simulink model "PEMFuelCellSystem_Cathode_cEGR_Focused_v01"  (R2025b)
settings: Solver=VariableStepAuto  StartTime=0.0  StopTime=100  MaxStep=0.1  RelTol=1e-3  AbsTol=1e-3
model workspace (MAT data in the model file):
  Gas_properties_block = 'PEMFuelCellSystem_Before_v01/Anode_Hydrogen_BOP/Gas Mixture
Properties'
  Gas_properties_candidates : object (value not decoded)
  T_TLU = [223.15 228.15 233.15 238.15 243.15 248.15 253.15 258.15 263.15 268.15 272.66 273.15 ... (115 elements, 1x115)]
  anode_separator_D = 0.02
  anode_separator_T0 = 20
  anode_separator_area = 0.000314159265359
  anode_separator_dp_nominal = 0.0005
  anode_separator_extra_length = 0.04
  anode_separator_laminar_fraction = 0.001
  anode_separator_length = 0.12
  anode_separator_mdot_nominal = 0.01
  anode_separator_p0 = 0.101325
  anode_separator_roughness = 1.5e-05
  anode_tube_D = 0.02
  cathode_outlet_chamber_V = 0.2
  cathode_separator_D = 0.05
  cathode_separator_T0 = 20
  cathode_separator_area = 0.00196349540849
  cathode_separator_dp_nominal = 0.0005
  cathode_separator_extra_length = 0.05
  cathode_separator_laminar_fraction = 0.001
  cathode_separator_length = 0.15
  cathode_separator_mdot_nominal = 0.1
  cathode_separator_p0 = 0.101325
  cathode_separator_roughness = 1.5e-05
  cathode_tube_D = 0.05
  cegr_comp_map_t_denom_epsilon = 1e-09
  cegr_cond_tau = 1
  cegr_inlet_mixer_p0 = 0.101325
  cegr_outlet_chamber_p0 = 0.101325
  cegr_pipe_D = 0.05
  cegr_pipe_area = 0.00196349540849
  cegr_pipe_extra_length = 0.1
  cegr_pipe_length = 0.5
  cegr_pipe_p0 = 0.101325
  cegr_pipe_roughness = 1.5e-05
  cegr_valve_max_area = 0.000196349540849
  cegr_valve_open_min_area = 1e-10
  comp_inlet_mixer_V = 0.1
  comp_mdot_corr_TLU = [0 0 0 0 0 0.2 0.15 0.1 0.05 0 0.4 0.3 ... (15 elements, 5x3)]
  comp_p_ratio_TLU = [1 1.25 1.5 1.75 2]
  comp_rpm_TLU = [0 1800 3600]
  coolant_num_layers = 20
  coolant_num_passes = 12
  coolant_tube_D = 0.05
  coolant_w_channels = 1
  drive_cycle_current = [0 0 100 100]
  drive_cycle_power = [0 0 40 40]
  drive_cycle_time = [0 0.5 60.5 600]
  drive_cycle_voltage = [427.6 427.6 410 410]
  env_RH = 0.5
  env_T = 20
  env_p = 0.101325
  env_pSat_H2O = 0.00233931818334
  env_yH20 = 0.0115436377169
  env_yO2 = 0.21
  focused_anode_boundary_T_C = 20
  focused_anode_feed_p_MPa_abs = 0.3
  focused_anode_inlet_mdot_kg_s = 0.001
  focused_anode_inlet_p_MPa_abs = 0.161325
  focused_anode_outlet_p_MPa_abs = 0.101325
  focused_anode_pipe_area = 0.000314159265359
  focused_anode_pipe_extra_length = 0.1
  focused_anode_pipe_length = 1
  focused_anode_pipe_roughness = 1.5e-05
  focused_anode_yH2 = 0.9997
  focused_stack_temperature_C = 80
  humidifier_bypass_mode : string (value not decoded)
  intercooler_Dh = 0.05
  intercooler_T0 = 20
  intercooler_area = 0.00196349540849
  intercooler_cond_tau = 1
  intercooler_dp_nominal = 0.001
  intercooler_extra_length = 0.05
  intercooler_laminar_fraction = 0.001
  intercooler_length = 0.25
  intercooler_mdot_nominal = 0.1
  intercooler_p0 = 0.101325
  intercooler_roughness = 1.5e-05
  pSat_H2O_TLU = [0.0039376926592 0.00720321689378 0.0128411282011 0.0223441068076 0.0380050105363 0.0632733889962 0.103238678713 0.165273175188 0.259872929049 0.401739659013 0.586936061043 0.611151401419 ... (115 elements, 1x115)]
  pSat_TLU = [3379.45709837 5023.40410987 1277.63968517 0.0039376926592 3379.45809837 5023.40510987 1277.64068517 0.00720321689378 3379.45909837 5023.40610987 1277.64168517 0.0128411282011 ... (460 elements, 4x115)]
  radiator_H = 0.5
  radiator_L = 1
  radiator_N_fins = 12000
  radiator_N_tubes = 25
  radiator_W = 0.025
  radiator_air_area_fins = 11.5625
  radiator_air_area_primary = 1.223125
  radiator_cp = 910
  radiator_eta_fin = 0.7
  radiator_fin_spacing = 0.002
  radiator_gap_H = 0.0192708333333
  radiator_rho = 2700
  radiator_t_wall = 0.0001
  radiator_tube_H = 0.0015
  radiator_tube_Leq = 2.5
  routeA_air_control_mode_id = 2
  routeA_air_pid_Ki = 0.5
  routeA_air_pid_Kp = 5
  routeA_anode_inlet_pressure_MPa_abs = 0.161325
  routeA_anode_purge_enable = 1
  routeA_anode_purge_off_n2_mole_fraction = 0.1
  routeA_anode_purge_on_n2_mole_fraction = 0.5
  routeA_anode_recirculation_base_command = 0.2
  routeA_anode_recirculation_current_gain_A_inv = 0.00204081632653
  routeA_anode_rh_setpoint = 1
  routeA_backpressure_control_mode_id = 1
  routeA_cathode_humidifier_gain = 1
  routeA_cathode_rh_setpoint = 1
  routeA_cegr_enabled = 1
  routeA_cegr_valve_mode_id = 1
  routeA_command_profile = [0 0.5 60.5 600 0.101325 0.101325 0.101325 0.101325 20 20 20 20 ... (92 elements, 4x23)]
  routeA_command_profile_baseline = [0.101325 20 0.21 0.0115436377169 0.045 3 0.5 0.1613 1 1 0 70 ... (22 elements, 1x22)]
  routeA_command_profile_fields : string (value not decoded)
  routeA_command_profile_schema : string (value not decoded)
  routeA_current_default_ref_A = 28
  routeA_egr_control_Ki_area = 3.92699081699e-05
  routeA_egr_control_Kp_area = 0.000196349540849
  routeA_egr_control_mode_id = 1
  routeA_egr_target_input_mode_id = 1
  routeA_egr_valve_actuator_tau = 0.5
  routeA_egr_valve_area_direct = 3.92699081699e-06
  routeA_external_case_enabled = 0
  routeA_parameter_layer : string (value not decoded)
  routeA_stack_temperature_set_C = 80
  routeA_target_egr_ratio_comp_in = 0.02
  routeA_voltage_current_max_A = 392
  routeA_voltage_current_min_A = 0
  routeA_voltage_default_ref_V = 394.9
  routeA_voltage_pi_Ki = 0.05
  routeA_voltage_pi_Kp = 1
  separator_condensation_enabled = 1
  separator_l2_efficiency = 0.5
  separator_l2_source : string (value not decoded)
  stack_alpha = 0.7
  stack_area = 280
  stack_iL = 1.4
  stack_io = 0.0001
  stack_mea_cp = 870
  stack_mea_rho = 1800
  stack_num_cells = 400
  stack_num_channels = 8
  stack_t_gdl = 250
  stack_t_membrane = 125
  stack_w_channels = 1
  tank_T = 20
  tank_V = 120
  tank_p = 70
  tank_yH2 = 0.9997
libraries: FuelCell_lib x43, fl_lib x34, nesl_utility x33, slpidlib x4
(part 3 of 4)

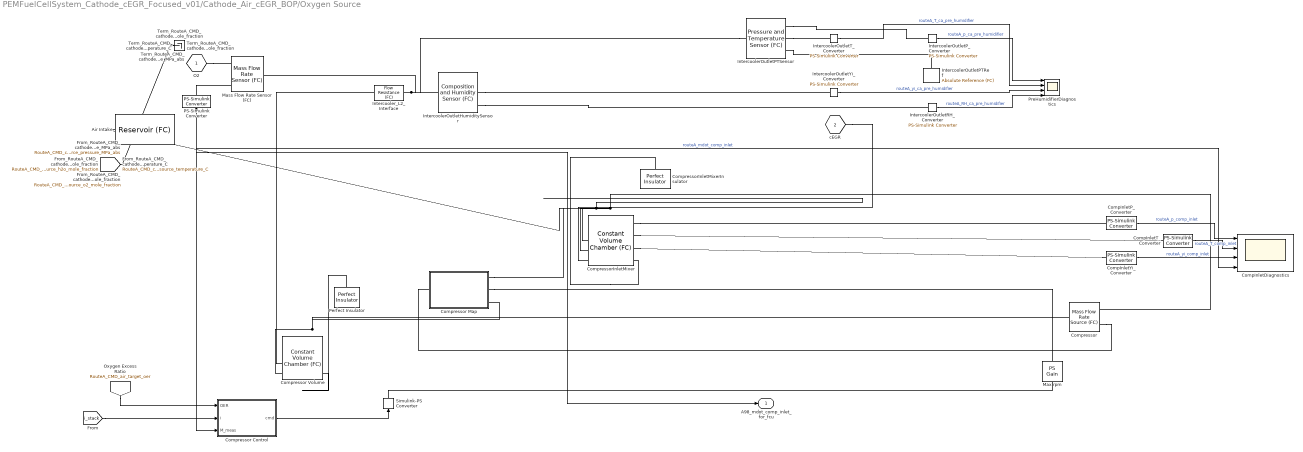
== system PEMFuelCellSystem_Cathode_cEGR_Focused_v01/Cathode_Air_cEGR_BOP/Oxygen Source ==
  Air Intake : FuelCell_lib/elements/Reservoir (FC)  constCond=true  p0=env_p MPa  T0=env_T degC  comp=FuelCell.enum.Composition.Mole  y0=[1-env_yO2-env_yH20; env_yO2; 0; env_yH20]  x0=[1; 0; 0; 0]  area=0.01 m^2
      settings: InternalSimscapePortConfiguration="{\"Bottom\":[],\"Left\":[],\"Right\":[],\"Top\":[{\"id\":\"A\",\"label\":\"A\",\"type\":\"FuelCell.FuelCell\"}]}"
  CompInletDiagnostics : Scope  NumInputPorts=4
  CompInletP_Converter : nesl_utility/PS-Simulink Converter  PhysicalDomain=network_engine_domain  SubClassName=ps_output  LeftPortType=input  RightPortType=output  PseudoPeriodic=off  Frequencies=[]  VectorFormat=inherit  Unit=inherit  AffineConversion=off
  CompInletT_Converter : nesl_utility/PS-Simulink Converter  PhysicalDomain=network_engine_domain  SubClassName=ps_output  LeftPortType=input  RightPortType=output  PseudoPeriodic=off  Frequencies=[]  VectorFormat=inherit  Unit=inherit  AffineConversion=off
  CompInletYi_Converter : nesl_utility/PS-Simulink Converter  PhysicalDomain=network_engine_domain  SubClassName=ps_output  LeftPortType=input  RightPortType=output  PseudoPeriodic=off  Frequencies=[]  VectorFormat=inherit  Unit=inherit  AffineConversion=off
  Compressor : FuelCell_lib/sources/Mass Flow Rate Source (FC)  source_type=foundation.enum.constant_controlled.controlled  flow_rate=0 kg/s  power_spec=foundation.enum.power_spec.isentropic  area_A=pi*cathode_tube_D^2/4 m^2  area_B=pi*cathode_tube_D^2/4 m^2  mdot_A_specify=off  mdot_A_priority=None  mdot_A=0.1 kg/s  mdot_A_nominal_specify=off  mdot_A_nominal_value=1  mdot_A_nominal_unit=kg/s  mdot_B_specify=off  mdot_B_priority=None  mdot_B=0.1 kg/s  mdot_B_nominal_specify=off  mdot_B_nominal_value=1  mdot_B_nominal_unit=kg/s  phi_A_specify=off  phi_A_priority=None  phi_A=0 J/s  phi_A_nominal_specify=off  phi_A_nominal_value=1  phi_A_nominal_unit=J/s  phi_B_specify=off  phi_B_priority=None  phi_B=0 J/s  phi_B_nominal_specify=off  phi_B_nominal_value=1  phi_B_nominal_unit=J/s  mdot_A_i_specify=off  mdot_A_i_priority=None  mdot_A_i=[0; 0; 0; 0] kg/s  mdot_A_i_nominal_specify=off  mdot_A_i_nominal_value=1  mdot_A_i_nominal_unit=kg/s  mdot_B_i_specify=off  mdot_B_i_priority=None  mdot_B_i=[0; 0; 0; 0] kg/s  mdot_B_i_nominal_specify=off  mdot_B_i_nominal_value=1  mdot_B_i_nominal_unit=kg/s
      settings: InternalSimscapePortConfiguration="{\"Bottom\":[],\"Left\":[{\"id\":\"M\",\"label\":\"M\",\"type\":\"input\"},{\"id\":\"A\",\"label\":\"A\",\"type\":\"FuelCell.FuelCell\"}],\"Right\":[{\"id\":\"B\",\"label\":\"B\",\"type\":\"FuelCell.FuelCell\"}],\"Top\":[]}"
  Compressor Volume : FuelCell_lib/elements/Constant Volume Chamber (FC)  V0=0.3 l  num_ports=foundation.enum.num_ports.two  area_A=pi*cathode_tube_D^2/4 m^2  area_B=pi*cathode_tube_D^2/4 m^2  area_C=0.01 m^2  area_D=0.01 m^2  cond_spec=FuelCell.enum.ChamberCondSpec.Enabled  tau_c=1e-3 s  is_cond=[0; 0; 0; 0]  out_comp=FuelCell.enum.Composition.Mole  p0=env_p MPa  T0=env_T degC  comp=FuelCell.enum.Composition.Mole  y0=[1-env_yO2-env_yH20; env_yO2; 0; env_yH20]  x0=[1; 0; 0; 0]
      settings: InternalSimscapePortConfiguration="{\"Bottom\":[{\"id\":\"H\",\"label\":\"H\",\"type\":\"foundation.thermal.thermal\"}],\"Left\":[{\"id\":\"MIn\",\"label\":\"MIn\",\"type\":\"input\"},{\"id\":\"TIn\",\"label\":\"TIn\",\"type\":\"input\"}],\"Right\":[{\"id\":\"pC\",\"label\":\"p\",\"type\":\"output\"},{\"id\":\"TC\",\"label\":\"T\",\"type\":\"output\"},{\"id\":\"yC_i\",\"label\":\"y_i\",\"type\":\"output\"}],\"Top\":[{\"id\":\"A\",\"label\":\"A\",\"type\":\"FuelCell.FuelCell\"},{\"id\":\"B\",\"label\":\"B\",\"type\":\"FuelCell.FuelCell\"}]}"
  Compressor Control : Subsystem
  Compressor Map : Subsystem
  CompressorInletMixer : FuelCell_lib/elements/Constant Volume Chamber (FC)  V0=comp_inlet_mixer_V l  num_ports=foundation.enum.num_ports.three  area_A=cegr_pipe_area m^2  area_B=cegr_pipe_area m^2  area_C=cegr_pipe_area m^2  area_D=0.01 m^2  cond_spec=FuelCell.enum.ChamberCondSpec.Enabled  tau_c=cegr_cond_tau s  is_cond=[0; 0; 0; 1]  out_comp=FuelCell.enum.Composition.Mole  p0=cegr_inlet_mixer_p0 MPa  T0=env_T degC  comp=FuelCell.enum.Composition.Mole  y0=[1-env_yO2-env_yH20; env_yO2; 0; env_yH20]  x0=[1; 0; 0; 0]
      settings: InternalSimscapePortConfiguration="{\"Bottom\":[{\"id\":\"H\",\"label\":\"H\",\"type\":\"foundation.thermal.thermal\"}],\"Left\":[{\"id\":\"MIn\",\"label\":\"MIn\",\"type\":\"input\"},{\"id\":\"TIn\",\"label\":\"TIn\",\"type\":\"input\"}],\"Right\":[{\"id\":\"pC\",\"label\":\"p\",\"type\":\"output\"},{\"id\":\"TC\",\"label\":\"T\",\"type\":\"output\"},{\"id\":\"yC_i\",\"label\":\"y_i\",\"type\":\"output\"}],\"Top\":[{\"id\":\"A\",\"label\":\"A\",\"type\":\"FuelCell.FuelCell\"},{\"id\":\"B\",\"label\":\"B\",\"type\":\"FuelCell.FuelCell\"},{\"id\":\"C\",\"label\":\"C\",\"type\":\"FuelCell.FuelCell\"}]}"
  CompressorInletMixerInsulator : fl_lib/Thermal/Thermal Elements/Perfect Insulator  T_specify=off  T_priority=None  T=env_T degC  T_nominal_specify=off  T_nominal_value=1  T_nominal_unit=K
  IntercoolerOutletHumiditySensor : FuelCell_lib/sensors/Composition and Humidity Sensor (FC)
      settings: InternalSimscapePortConfiguration="{\"Bottom\":[],\"Left\":[{\"id\":\"A\",\"label\":\"A\",\"type\":\"FuelCell.FuelCell\"}],\"Right\":[{\"id\":\"x_i\",\"label\":\"x_i\",\"type\":\"output\"},{\"id\":\"y_i\",\"label\":\"y_i\",\"type\":\"output\"},{\"id\":\"W\",\"label\":\"W\",\"type\":\"output\"}],\"Top\":[]}"
  IntercoolerOutletPTRef : FuelCell_lib/elements/Absolute Reference (FC)
      settings: InternalSimscapePortConfiguration="{\"Bottom\":[],\"Left\":[{\"id\":\"A\",\"label\":\"\",\"type\":\"FuelCell.FuelCell\"}],\"Right\":[],\"Top\":[]}"
  IntercoolerOutletPTSensor : FuelCell_lib/sensors/Pressure and Temperature Sensor (FC)
      settings: InternalSimscapePortConfiguration="{\"Bottom\":[],\"Left\":[{\"id\":\"A\",\"label\":\"A\",\"type\":\"FuelCell.FuelCell\"}],\"Right\":[{\"id\":\"P\",\"label\":\"P\",\"type\":\"output\"},{\"id\":\"T\",\"label\":\"T\",\"type\":\"output\"},{\"id\":\"B\",\"label\":\"B\",\"type\":\"FuelCell.FuelCell\"}],\"Top\":[]}"
  IntercoolerOutletP_Converter : nesl_utility/PS-Simulink Converter  PhysicalDomain=network_engine_domain  SubClassName=ps_output  LeftPortType=input  RightPortType=output  PseudoPeriodic=off  Frequencies=[]  VectorFormat=inherit  Unit=inherit  AffineConversion=off
  IntercoolerOutletRH_Converter : nesl_utility/PS-Simulink Converter  PhysicalDomain=network_engine_domain  SubClassName=ps_output  LeftPortType=input  RightPortType=output  PseudoPeriodic=off  Frequencies=[]  VectorFormat=inherit  Unit=inherit  AffineConversion=off
  IntercoolerOutletT_Converter : nesl_utility/PS-Simulink Converter  PhysicalDomain=network_engine_domain  SubClassName=ps_output  LeftPortType=input  RightPortType=output  PseudoPeriodic=off  Frequencies=[]  VectorFormat=inherit  Unit=inherit  AffineConversion=off
  IntercoolerOutletYi_Converter : nesl_utility/PS-Simulink Converter  PhysicalDomain=network_engine_domain  SubClassName=ps_output  LeftPortType=input  RightPortType=output  PseudoPeriodic=off  Frequencies=[]  VectorFormat=inherit  Unit=inherit  AffineConversion=off
  Intercooler_L2_Interface : FuelCell_lib/elements/Flow Resistance (FC)  var_res=false  delta_p_nominal=intercooler_dp_nominal MPa  mdot_nominal=intercooler_mdot_nominal kg/s  rho_nominal=0 kg/m^3  laminar_fraction=intercooler_laminar_fraction  area=intercooler_area m^2  leak_thresh=1e-5
      settings: InternalSimscapePortConfiguration="{\"Bottom\":[],\"Left\":[{\"id\":\"A\",\"label\":\"A\",\"type\":\"FuelCell.FuelCell\"}],\"Right\":[{\"id\":\"B\",\"label\":\"B\",\"type\":\"FuelCell.FuelCell\"}],\"Top\":[]}"
  Mass Flow Rate Sensor (FC) : FuelCell_lib/sensors/Mass Flow Rate Sensor (FC)
      settings: InternalSimscapePortConfiguration="{\"Bottom\":[],\"Left\":[{\"id\":\"A\",\"label\":\"A\",\"type\":\"FuelCell.FuelCell\"}],\"Right\":[{\"id\":\"M\",\"label\":\"M\",\"type\":\"output\"},{\"id\":\"Phi_out\",\"label\":\"Phi\",\"type\":\"output\"},{\"id\":\"M_i\",\"label\":\"M_i\",\"type\":\"output\"},{\"id\":\"B\",\"label\":\"B\",\"type\":\"FuelCell.FuelCell\"}],\"Top\":[]}"
  Max rpm : fl_lib/Physical Signals/Functions/PS Gain  gain=max(comp_rpm_TLU) rpm
  PS-Simulink Converter : nesl_utility/PS-Simulink Converter  PhysicalDomain=network_engine_domain  SubClassName=ps_output  LeftPortType=input  RightPortType=output  PseudoPeriodic=off  Frequencies=[]  VectorFormat=1-D array  Unit=kg/s  AffineConversion=off
  Perfect Insulator : fl_lib/Thermal/Thermal Elements/Perfect Insulator  T_specify=off  T_priority=None  T=env_T degC  T_nominal_specify=off  T_nominal_value=1  T_nominal_unit=K
  PreHumidifierDiagnostics : Scope  NumInputPorts=4
  Simulink-PS Converter : nesl_utility/Simulink-PS Converter  PhysicalDomain=network_engine_domain  SubClassName=ps_input  LeftPortType=input  RightPortType=output  PseudoPeriodic=off  Frequencies=[]  NoiseDistribution=none  NoiseParameters=[]  Unit=1  AffineConversion=off  FilteringAndDerivatives=provide  SimscapeFilterOrder=1  InputFilterTimeConstant=0.001  UdotUserProvided=0
  Term_RouteA_CMD_cathode_source_h2o_mole_fraction : Terminator
  Term_RouteA_CMD_cathode_source_o2_mole_fraction : Terminator
  Term_RouteA_CMD_cathode_source_pressure_MPa_abs : Terminator
  Term_RouteA_CMD_cathode_source_temperature_C : Terminator
  O2 : PMIOPort  Side=Left
  cEGR : PMIOPort  Port=2  Side=Left
  A98_mdot_comp_inlet_for_fcu : Outport
  wires:
  CompInletT_Converter/1 -> CompInletDiagnostics/2  "routeA_T_comp_inlet"
  CompInletP_Converter/1 -> CompInletDiagnostics/1  "routeA_p_comp_inlet"
  Compressor Control/1(cmd) -> Simulink-PS Converter/1
  [i_stack] -> Compressor Control/2(i)
  CompInletYi_Converter/1 -> CompInletDiagnostics/3  "routeA_yi_comp_inlet"
  PS-Simulink Converter/1 -> A98_mdot_comp_inlet_for_fcu/1, Compressor Control/3(M_meas), CompInletDiagnostics/4  "routeA_mdot_comp_inlet"
  IntercoolerOutletP_Converter/1 -> PreHumidifierDiagnostics/1  "routeA_p_ca_pre_humidifier"
  IntercoolerOutletT_Converter/1 -> PreHumidifierDiagnostics/2  "routeA_T_ca_pre_humidifier"
  IntercoolerOutletYi_Converter/1 -> PreHumidifierDiagnostics/3  "routeA_yi_ca_pre_humidifier"
  IntercoolerOutletRH_Converter/1 -> PreHumidifierDiagnostics/4  "routeA_RH_ca_pre_humidifier"
  [RouteA_CMD_air_target_oer] -> Compressor Control/1(OER)
  [RouteA_CMD_cathode_source_o2_mole_fraction] -> Term_RouteA_CMD_cathode_source_o2_mole_fraction/1
  [RouteA_CMD_cathode_source_h2o_mole_fraction] -> Term_RouteA_CMD_cathode_source_h2o_mole_fraction/1
  [RouteA_CMD_cathode_source_pressure_MPa_abs] -> Term_RouteA_CMD_cathode_source_pressure_MPa_abs/1
  [RouteA_CMD_cathode_source_temperature_C] -> Term_RouteA_CMD_cathode_source_temperature_C/1
  connections:
  CompressorInletMixer/LConn3 -- Air Intake/LConn1
  IntercoolerOutletHumiditySensor/RConn3 -- IntercoolerOutletRH_Converter/LConn1
  IntercoolerOutletHumiditySensor/RConn2 -- IntercoolerOutletYi_Converter/LConn1
  IntercoolerOutletPTSensor/RConn2 -- IntercoolerOutletT_Converter/LConn1
  IntercoolerOutletPTSensor/RConn1 -- IntercoolerOutletP_Converter/LConn1
  IntercoolerOutletPTSensor/LConn1 -- Intercooler_L2_Interface/RConn1 -- Mass Flow Rate Sensor (FC)/LConn1 -- IntercoolerOutletHumiditySensor/LConn1
  Compressor/LConn1 -- Compressor Map/LConn1
  CompressorInletMixer/RConn2 -- CompInletT_Converter/LConn1
  CompressorInletMixer/RConn1 -- CompInletP_Converter/LConn1
  Compressor Map/RConn2 -- Max rpm/RConn1
  CompressorInletMixer/LConn4 -- Compressor Map/RConn1 -- Compressor/LConn2
  cEGR/RConn1 -- CompressorInletMixer/LConn5
  Simulink-PS Converter/RConn1 -- Max rpm/LConn1
  CompressorInletMixer/RConn3 -- CompInletYi_Converter/LConn1
  Compressor Map/RConn3 -- Compressor Volume/LConn4 -- Compressor/RConn1
  CompressorInletMixerInsulator/LConn1 -- CompressorInletMixer/RConn4
  Perfect Insulator/LConn1 -- Compressor Volume/RConn4
  PS-Simulink Converter/LConn1 -- Mass Flow Rate Sensor (FC)/RConn1
  O2/RConn1 -- Mass Flow Rate Sensor (FC)/RConn4
  IntercoolerOutletPTSensor/RConn3 -- IntercoolerOutletPTRef/LConn1
  Intercooler_L2_Interface/LConn1 -- Compressor Volume/LConn3

== system PEMFuelCellSystem_Cathode_cEGR_Focused_v01/Cathode_Exhaust_Backpressure_Water/Cathode Exhaust ==
  Constant1 : Constant  Value=0
  Convective Heat Transfer1 : fl_lib/Thermal/Thermal Elements/Convective Heat Transfer  thermal_type=foundation.enum.constant_variable.constant  area=pi*cathode_tube_D*1 m^2  heat_tr_coeff=20 W/(m^2 * K)  min_heat_tr_coeff=1e-3 W/(K*m^2)  T_specify=off  T_priority=None  T=0 K  T_nominal_specify=off  T_nominal_value=1  T_nominal_unit=K  Q_specify=off  Q_priority=None  Q=0 W  Q_nominal_specify=off  Q_nominal_value=1  Q_nominal_unit=W
  Environment : FuelCell_lib/elements/Reservoir (FC)  constCond=true  p0=env_p MPa  T0=env_T degC  comp=FuelCell.enum.Composition.Mole  y0=[1-env_yO2-env_yH20; env_yO2; 0; env_yH20]  x0=[1; 0; 0; 0]  area=pi*cathode_tube_D^2/4 m^2
      settings: InternalSimscapePortConfiguration="{\"Bottom\":[],\"Left\":[],\"Right\":[],\"Top\":[{\"id\":\"A\",\"label\":\"A\",\"type\":\"FuelCell.FuelCell\"}]}"
  Environment Temperature : fl_lib/Thermal/Thermal Sources/Temperature Source  temperature=env_T degC
  Pipe (N Gas)1 : FuelCell_lib/elements/Pipe (FC)  length=1 m  area=pi*cathode_tube_D^2/4 m^2  Dh=cathode_tube_D m  extra_length=0.1 m  roughness=15e-6 m  Re_lam=2000  Re_tur=4000  shape_factor=64  Nu_lam=3.66  tau_c=1e-3 s  isCond=[0; 0; 0; 0]  volMeas=false  compMeas=FuelCell.enum.Composition.Mole  p0=env_p MPa  T0=env_T degC  comp=FuelCell.enum.Composition.Mole  y0=[1-env_yO2-env_yH20; env_yO2; 0; env_yH20]  x0=[1; 0; 0; 0]
      settings: InternalSimscapePortConfiguration="{\"Bottom\":[{\"id\":\"MIn\",\"label\":\"M_in\",\"type\":\"input\"},{\"id\":\"TIn\",\"label\":\"T_in\",\"type\":\"input\"}],\"Left\":[{\"id\":\"A\",\"label\":\"A\",\"type\":\"FuelCell.FuelCell\"},{\"id\":\"H\",\"label\":\"H\",\"type\":\"foundation.thermal.thermal\"}],\"Right\":[{\"id\":\"B\",\"label\":\"B\",\"type\":\"FuelCell.FuelCell\"}],\"Top\":[]}"
  Pressure Relief Valve : Subsystem  Tag=PublishSubsystem  mask(Pressure Relief Valve){D=cathode_tube_D, r_min=1e-4, r_max=0.8, p_range=0.005}
      mask prompts: D "Connecting tube diameter (m)"; r_min "Min diameter ratio"; r_max "Max diameter ratio"; p_range "Pressure regulation range (MPa)"
      mask help: This subsystem models a pressure relief valve that maintains a set pressure at port A. The valve is normally closed. When the pressure is above the set pressure, it begins to open.
  Simulink-PS Converter1 : nesl_utility/Simulink-PS Converter  PhysicalDomain=network_engine_domain  SubClassName=ps_input  LeftPortType=input  RightPortType=output  PseudoPeriodic=off  Frequencies=[]  NoiseDistribution=none  NoiseParameters=[]  Unit=MPa  AffineConversion=off  FilteringAndDerivatives=provide  SimscapeFilterOrder=1  InputFilterTimeConstant=0.001  UdotUserProvided=0
  Sum : Sum  Inputs=++|
  C : PMIOPort  Side=Left
  wires:
  Sum/1 -> Simulink-PS Converter1/1
  Constant1/1 -> Sum/2
  [RouteA_CMD_cathode_outlet_pressure_MPa_abs] -> Sum/1
  connections:
  C/RConn1 -- Pipe (N Gas)1/LConn1
  Simulink-PS Converter1/RConn1 -- Pressure Relief Valve/LConn2
  Pipe (N Gas)1/RConn1 -- Pressure Relief Valve/LConn1
  Pressure Relief Valve/RConn1 -- Environment/LConn1
  Convective Heat Transfer1/LConn1 -- Pipe (N Gas)1/LConn2
  Environment Temperature/LConn1 -- Convective Heat Transfer1/RConn1

== system PEMFuelCellSystem_Cathode_cEGR_Focused_v01/Stack_Core/Anode Gas Channels ==
  Anode : FuelCell_lib/elements/Constant Volume Chamber (FC)  V0=stack_w_channels^2 * stack_num_channels * stack_num_cells * sqrt(stack_area) cm^3  num_ports=foundation.enum.num_ports.three  area_A=stack_w_channels^2 * stack_num_channels * stack_num_cells cm^2  area_B=stack_w_channels^2 * stack_num_channels * stack_num_cells cm^2  area_C=stack_w_channels^2 * stack_num_channels * stack_num_cells cm^2  area_D=0.01 m^2  cond_spec=FuelCell.enum.ChamberCondSpec.Enabled  tau_c=1e-3 s  is_cond=[0; 0; 0; 0]  out_comp=FuelCell.enum.Composition.Mass  p0=env_p MPa  T0=env_T degC  comp=FuelCell.enum.Composition.Mole  y0=[0; 0; 1; 0]  x0=[1; 0; 0; 0]
      settings: InternalSimscapePortConfiguration="{\"Bottom\":[{\"id\":\"H\",\"label\":\"H\",\"type\":\"foundation.thermal.thermal\"}],\"Left\":[{\"id\":\"MIn\",\"label\":\"MIn\",\"type\":\"input\"},{\"id\":\"TIn\",\"label\":\"TIn\",\"type\":\"input\"}],\"Right\":[{\"id\":\"pC\",\"label\":\"p\",\"type\":\"output\"},{\"id\":\"TC\",\"label\":\"T\",\"type\":\"output\"},{\"id\":\"xC_i\",\"label\":\"x_i\",\"type\":\"output\"}],\"Top\":[{\"id\":\"A\",\"label\":\"A\",\"type\":\"FuelCell.FuelCell\"},{\"id\":\"B\",\"label\":\"B\",\"type\":\"FuelCell.FuelCell\"},{\"id\":\"C\",\"label\":\"C\",\"type\":\"FuelCell.FuelCell\"}]}"
  A : PMIOPort  Side=Right
  Min : PMIOPort  Port=2  Side=Right
  Tin : PMIOPort  Port=3  Side=Right
  H : PMIOPort  Port=4  Side=Right
  B : PMIOPort  Port=5  Side=Left
  C : PMIOPort  Port=6  Side=Left
  xi : PMIOPort  Port=7  Side=Left
  connections:
  B/RConn1 -- Anode/LConn4
  Min/RConn1 -- Anode/LConn1
  Tin/RConn1 -- Anode/LConn2
  xi/RConn1 -- Anode/RConn3
  Anode/LConn5 -- C/RConn1
  A/RConn1 -- Anode/LConn3
  H/RConn1 -- Anode/RConn4

== system PEMFuelCellSystem_Cathode_cEGR_Focused_v01/Stack_Core/Cathode Gas Channels ==
  Cathode : FuelCell_lib/elements/Constant Volume Chamber (FC)  V0=stack_w_channels^2 * stack_num_channels * stack_num_cells * sqrt(stack_area) cm^3  num_ports=foundation.enum.num_ports.three  area_A=stack_w_channels^2 * stack_num_channels * stack_num_cells cm^2  area_B=stack_w_channels^2 * stack_num_channels * stack_num_cells cm^2  area_C=stack_w_channels^2 * stack_num_channels * stack_num_cells cm^2  area_D=0.01 m^2  cond_spec=FuelCell.enum.ChamberCondSpec.Enabled  tau_c=1e-3 s  is_cond=[0; 0; 0; 0]  out_comp=FuelCell.enum.Composition.Mass  p0=env_p MPa  T0=env_T degC  comp=FuelCell.enum.Composition.Mole  y0=[1-env_yO2-env_yH20; env_yO2; 0; env_yH20]  x0=[1; 0; 0; 0]
      settings: InternalSimscapePortConfiguration="{\"Bottom\":[{\"id\":\"H\",\"label\":\"H\",\"type\":\"foundation.thermal.thermal\"}],\"Left\":[{\"id\":\"MIn\",\"label\":\"MIn\",\"type\":\"input\"},{\"id\":\"TIn\",\"label\":\"TIn\",\"type\":\"input\"}],\"Right\":[{\"id\":\"pC\",\"label\":\"p\",\"type\":\"output\"},{\"id\":\"TC\",\"label\":\"T\",\"type\":\"output\"},{\"id\":\"xC_i\",\"label\":\"x_i\",\"type\":\"output\"}],\"Top\":[{\"id\":\"A\",\"label\":\"A\",\"type\":\"FuelCell.FuelCell\"},{\"id\":\"B\",\"label\":\"B\",\"type\":\"FuelCell.FuelCell\"},{\"id\":\"C\",\"label\":\"C\",\"type\":\"FuelCell.FuelCell\"}]}"
  A : PMIOPort  Side=Right
  Min : PMIOPort  Port=2  Side=Right
  Tin : PMIOPort  Port=3  Side=Right
  H : PMIOPort  Port=4  Side=Right
  B : PMIOPort  Port=5  Side=Left
  C : PMIOPort  Port=6  Side=Left
  xi : PMIOPort  Port=7  Side=Left
  connections:
  B/RConn1 -- Cathode/LConn4
  Min/RConn1 -- Cathode/LConn1
  Tin/RConn1 -- Cathode/LConn2
  xi/RConn1 -- Cathode/RConn3
  H/RConn1 -- Cathode/RConn4
  Cathode/LConn5 -- C/RConn1
  A/RConn1 -- Cathode/LConn3

== system PEMFuelCellSystem_Cathode_cEGR_Focused_v01/System_Control_Observability/Electrical Load ==
  Controlled Current Source : fl_lib/Electrical/Electrical Sources/Controlled Current Source
  Electrical Reference : fl_lib/Electrical/Electrical Elements/Electrical Reference
  Inputs : Subsystem  Variant=on  VariantControlMode=label  LabelModeActiveChoice=Voltage
      settings: PortSchema="{\"entries\":[{\"content\":{\"sides\":[{\"content\":{\"connectorIds\":[\"LConn1\"]},\"type\":\"ConnectorPlacement.EquallySpacedRectSide\",\"uuid\":\"316ab41f-9548-4c29-941b-82cd3006a9cc\"},{\"content\":{\"connectorIds\":[],\"side\":\"RIGHT\"},\"type\":\"ConnectorPlacement.EquallySpacedRectSide\",\"uuid\":\"21ddf6a1-5f8a-47a4-ab15-3c27c3a556ce\"},{\"content\":{\"connectorIds\":[\"LConn2\"],\"side\":\"TOP\"},\"type\":\"ConnectorPlacement.EquallySpacedRectSide\",\"uuid\":\"59191a52-f145-4ac2-9cf2-0e0b54b3d2a8\"}]},\"type\":\"ConnectorPlacement.EquallySpacedConnector\",\"uuid\":\"e8f988fd-b412-4b1a-aaea-374cf82170cc\"}],\"packageUris\":[\"http://schema.mathworks.com/mf0/Connector/R2020b\"],\"version\":\"1.0\"}"
      mask Display:
      | blk = get_param(gcb, 'CompiledActiveChoiceBlock');
      | eval(get_param(blk, 'MaskDisplay'))
  Voltage Sensor : fl_lib/Electrical/Electrical Sensors/Voltage Sensor
  - : PMIOPort  Side=Right
  + : PMIOPort  Port=2  Side=Right
  connections:
  Electrical Reference/LConn1 -- Controlled Current Source/LConn1 -- -/RConn1 -- Voltage Sensor/RConn2
  +/RConn1 -- Voltage Sensor/LConn1 -- Controlled Current Source/RConn2
  Voltage Sensor/RConn1 -- Inputs/LConn2
  Inputs/LConn1 -- Controlled Current Source/RConn1

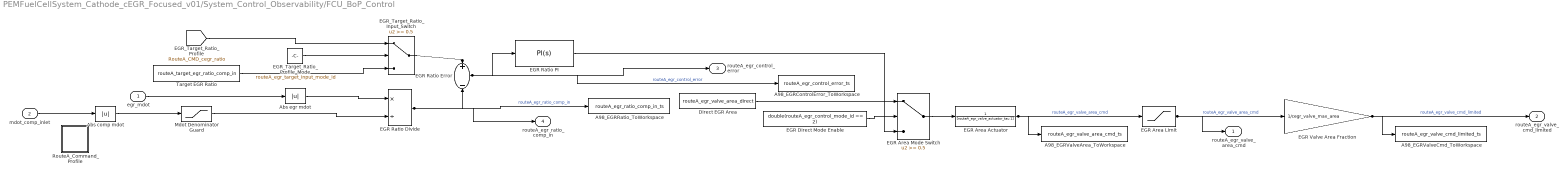
== system PEMFuelCellSystem_Cathode_cEGR_Focused_v01/System_Control_Observability/FCU_BoP_Control ==
  egr_mdot : Inport
  mdot_comp_inlet : Inport  Port=2
  A98_EGRControlError_ToWorkspace : ToWorkspace  VariableName=routeA_egr_control_error_ts  SaveFormat=Timeseries  SampleTime=-1
  A98_EGRRatio_ToWorkspace : ToWorkspace  VariableName=routeA_egr_ratio_comp_in_ts  SaveFormat=Timeseries  SampleTime=-1
  A98_EGRValveArea_ToWorkspace : ToWorkspace  VariableName=routeA_egr_valve_area_cmd_ts  SaveFormat=Timeseries  SampleTime=-1
  A98_EGRValveCmd_ToWorkspace : ToWorkspace  VariableName=routeA_egr_valve_cmd_limited_ts  SaveFormat=Timeseries  SampleTime=-1
  Abs comp mdot : Abs  ZeroCross=off  SaturateOnIntegerOverflow=off
  Abs egr mdot : Abs  ZeroCross=off  SaturateOnIntegerOverflow=off
  Direct EGR Area : Constant  Value=routeA_egr_valve_area_direct
  EGR Area Actuator : TransferFcn  Denominator=[routeA_egr_valve_actuator_tau 1]
  EGR Area Limit : Saturate  UpperLimit=cegr_valve_max_area  LowerLimit=cegr_valve_open_min_area
  EGR Area Mode Switch : Switch  Threshold=0.5  SaturateOnIntegerOverflow=off  InputSameDT=off
  EGR Direct Mode Enable : Constant  Value=double(routeA_egr_control_mode_id == 2)
  EGR Ratio Divide : Product  Inputs=*/
  EGR Ratio Error : Sum  Inputs=+-
  EGR Ratio PI : slpidlib/PID Controller  Controller=PI  Form=Parallel  TimeDomain=Continuous-time  UseExternalTs=off  SampleTime=-1  IntegratorMethod=Forward Euler  FilterMethod=Forward Euler  ControllerParametersSource=internal  P=routeA_egr_control_Kp_area  I=routeA_egr_control_Ki_area  UseKiTs=off  D=0  UseExternalDerivativeSource=off  N=100  UseFilter=on  TunerSelectOption=Transfer Function Based (PID Tuner App)  ZeroCross=off  InitialConditionSource=internal  InitialConditionForIntegrator=cegr_valve_open_min_area  InitialConditionForFilter=0  DifferentiatorICPrevScaledInput=0  ExternalReset=none  TrackingMode=off  Kt=1  LimitOutput=on  SatLimitsSource=internal  UpperSaturationLimit=cegr_valve_max_area  LowerSaturationLimit=cegr_valve_open_min_area  LinearizeAsGain=on  AntiWindupMode=none  Kb=1  LimitIntegrator=off  UpperIntegratorSaturationLimit=inf  LowerIntegratorSaturationLimit=-inf  POutMin=[]  POutMax=[]  IOutMin=[]  IOutMax=[]  DOutMin=[]  DOutMax=[]  NOutMin=[]  NOutMax=[]  SumOutMin=[]  SumOutMax=[]  SaturationOutMin=[]  SaturationOutMax=[]  PParamMin=[]  PParamMax=[]  IParamMin=[]  IParamMax=[]  DParamMin=[]  DParamMax=[]  NParamMin=[]  NParamMax=[]  KbParamMin=[]  KbParamMax=[]  KtParamMin=[]  KtParamMax=[]  KbOutMin=[]  KbOutMax=[]  KtOutMin=[]  KtOutMax=[]  IntegratorOutMin=[]  IntegratorOutMax=[]  FilterOutMin=[]  FilterOutMax=[]  SumI1OutMin=[]  SumI1OutMax=[]  SumI2OutMin=[]  SumI2OutMax=[]  SumI3OutMin=[]  SumI3OutMax=[]  SumI4OutMin=[]  SumI4OutMax=[]  SumDOutMin=[]  SumDOutMax=[]  DifferentiatorOutMin=[]  DifferentiatorOutMax=[]  FilterDiffOutCoefMin=[]  FilterDiffOutCoefMax=[]  ReciprocalOutMin=[]  ReciprocalOutMax=[]  SumDenOutMin=[]  SumDenOutMax=[]  SumNumOutMin=[]  SumNumOutMax=[]  DivideOutMin=[]  DivideOutMax=[]  UdiffTsProdOutMin=[]  UdiffTsProdOutMax=[]  NTsProdOutMin=[]  NTsProdOutMax=[]  UintegralTsProdOutMin=[]  UintegralTsProdOutMax=[]  UngainTsProdOutMin=[]  UngainTsProdOutMax=[]  ClampingZeroOutDataTypeStr=Inherit: Inherit via back propagation  ClampingZeroOutMin=[]  ClampingZeroOutMax=[]  FilterDenConstantOutDataTypeStr=Inherit: Inherit via back propagation  FilterDenConstantOutMin=[]  FilterDenConstantOutMax=[]  PCopyOutDataTypeStr=Inherit: Inherit via back propagation  PCopyOutMin=[]  PCopyOutMax=[]  NCopyOutDataTypeStr=Inherit: Inherit via back propagation  NCopyOutMin=[]  NCopyOutMax=[]  IntegratorContinuousStateAttributes=''  IntegratorStateMustResolveToSignalObject=off  IntegratorRTWStateStorageClass=Auto  FilterContinuousStateAttributes=''  FilterStateMustResolveToSignalObject=off  FilterRTWStateStorageClass=Auto  ParallelPVariant=InternalParameters  IdealPVariant=Disabled  IVariant=InternalParameters  DVariant=Disabled  IntegratorVariant=Continuous  SatVariant=Enabled  AWVariant=Passthrough  PCopyVariant=Disabled  TRVariant=Disabled  FdbkBlocksVariant=Forward  IdealPFdbkVariant=Disabled  SatFdbkVariant=Disabled  DerivativeFilterVariant=Disabled  NVariant=Disabled  NCopyVariant=Disabled_SignalSpec  FilterICVariant=Disabled  IntegratorICVariant=InternalICs  ExternalResetVariant=Disabled  TRSumVariant=Passthrough  SumFdbkVariant=Disabled  SumVariant=Sum_PI  TsampFilterVariant=InternalTs  TsampNgainVariant=Passthrough  TsampIntegralVariant=Disabled_SignalSpec  ExternalSaturationOutDataTypeStr=Inherit: Same as second input  DerivativeSourceVariant=Disabled  PreIntVariant=InternalPreInt
  EGR Valve Area Fraction : Gain  Gain=1/cegr_valve_max_area
  EGR_Target_Ratio_Input_Switch : Switch  Threshold=0.5
  EGR_Target_Ratio_Profile_Mode : Constant  Value=routeA_egr_target_input_mode_id
  Mdot Denominator Guard : Saturate  UpperLimit=inf  LowerLimit=1e-6
  RouteA_Command_Profile : Subsystem
  Target EGR Ratio : Constant  Value=routeA_target_egr_ratio_comp_in
  routeA_egr_valve_area_cmd : Outport
  routeA_egr_valve_cmd_limited : Outport  Port=2
  routeA_egr_control_error : Outport  Port=3
  routeA_egr_ratio_comp_in : Outport  Port=4
  wires:
  [RouteA_CMD_cegr_ratio] -> EGR_Target_Ratio_Input_Switch/1
  EGR_Target_Ratio_Input_Switch/1 -> EGR Ratio Error/1
  EGR_Target_Ratio_Profile_Mode/1 -> EGR_Target_Ratio_Input_Switch/2
  EGR Area Limit/1 -> EGR Valve Area Fraction/1, routeA_egr_valve_area_cmd/1  "routeA_egr_valve_area_cmd"
  EGR Area Actuator/1 -> EGR Area Limit/1, A98_EGRValveArea_ToWorkspace/1  "routeA_egr_valve_area_cmd"
  EGR Area Mode Switch/1 -> EGR Area Actuator/1
  EGR Ratio PI/1 -> EGR Area Mode Switch/3
  EGR Direct Mode Enable/1 -> EGR Area Mode Switch/2
  Direct EGR Area/1 -> EGR Area Mode Switch/1
  EGR Ratio Divide/1 -> routeA_egr_ratio_comp_in/1, A98_EGRRatio_ToWorkspace/1, EGR Ratio Error/2  "routeA_egr_ratio_comp_in"
  EGR Ratio Error/1 -> A98_EGRControlError_ToWorkspace/1, routeA_egr_control_error/1, EGR Ratio PI/1  "routeA_egr_control_error"
  Mdot Denominator Guard/1 -> EGR Ratio Divide/2
  Abs egr mdot/1 -> EGR Ratio Divide/1
  Target EGR Ratio/1 -> EGR_Target_Ratio_Input_Switch/3
  egr_mdot/1 -> Abs egr mdot/1
  Abs comp mdot/1 -> Mdot Denominator Guard/1
  EGR Valve Area Fraction/1 -> A98_EGRValveCmd_ToWorkspace/1, routeA_egr_valve_cmd_limited/1  "routeA_egr_valve_cmd_limited"
  mdot_comp_inlet/1 -> Abs comp mdot/1

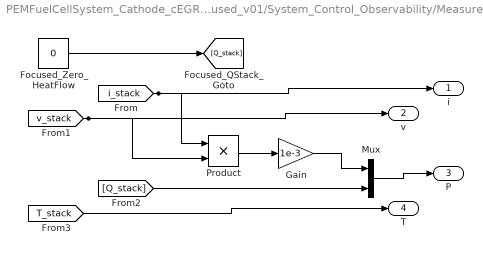
== system PEMFuelCellSystem_Cathode_cEGR_Focused_v01/System_Control_Observability/Measurements ==
  Focused_Zero_HeatFlow : Constant  Value=0
  Gain : Gain  Gain=1e-3
  Mux : Mux  Inputs=2
  Product : Product
  i : Outport
  v : Outport  Port=2
  P : Outport  Port=3
  T : Outport  Port=4
  wires:
  Focused_Zero_HeatFlow/1 -> [Q_stack]
  Gain/1 -> Mux/1
  Mux/1 -> P/1
  Product/1 -> Gain/1
  [Q_stack] -> Mux/2
  [T_stack] -> T/1
  [i_stack] -> i/1, Product/1
  [v_stack] -> v/1, Product/2

== system PEMFuelCellSystem_Cathode_cEGR_Focused_v01/cEGR_Mode_Selector/noCEGR_Isolation ==
  NoCEGR_CathodeIsolation : FuelCell_lib/elements/Infinite Flow Resistance (FC)  p_specify=off  p_priority=None  p=0 MPa  p_nominal_specify=off  p_nominal_value=1  p_nominal_unit=MPa  T_specify=off  T_priority=None  T=0 K  T_nominal_specify=off  T_nominal_value=1  T_nominal_unit=K  x_i_specify=off  x_i_priority=None  x_i=[0; 0; 0; 0]  x_i_nominal_specify=off  x_i_nominal_value=1  x_i_nominal_unit=1
      settings: InternalSimscapePortConfiguration="{\"Bottom\":[],\"Left\":[{\"id\":\"A\",\"label\":\"A\",\"type\":\"FuelCell.FuelCell\"}],\"Right\":[{\"id\":\"B\",\"label\":\"B\",\"type\":\"FuelCell.FuelCell\"}],\"Top\":[]}"
  A : PMIOPort  Side=Left
  B : PMIOPort  Port=2  Side=Left
  connections:
  A/RConn1 -- NoCEGR_CathodeIsolation/LConn1
  NoCEGR_CathodeIsolation/RConn1 -- B/RConn1

== system PEMFuelCellSystem_Cathode_cEGR_Focused_v01/cEGR_Mode_Selector/withCEGR_PassThrough ==
  A : PMIOPort  Side=Left
  B : PMIOPort  Port=2  Side=Left
  connections:
  A/RConn1 -- B/RConn1

== system PEMFuelCellSystem_Cathode_cEGR_Focused_v01/Cathode_Air_cEGR_BOP/Cathode Humidifier/Proportional Control ==
  RH_set : Inport
  RH_meas : Inport  Port=2
  Gain : Gain  Gain=0.1
  Saturation : Saturate  UpperLimit=inf  LowerLimit=0  ZeroCross=off
  Selector : Selector  InputPortWidth=4  IndexOptions=Index vector (dialog)  Indices=[4]  OutputSizes=1
  Sum : Sum  Inputs=|+-
  Transfer Fcn : TransferFcn  Denominator=[1 1]
  Mw : Outport
  wires:
  Saturation/1 -> Transfer Fcn/1
  Gain/1 -> Saturation/1
  Transfer Fcn/1 -> Mw/1
  RH_meas/1 -> Selector/1
  Sum/1 -> Gain/1
  RH_set/1 -> Sum/1
  Selector/1 -> Sum/2

== system PEMFuelCellSystem_Cathode_cEGR_Focused_v01/Cathode_Air_cEGR_BOP/EGRValveRestriction/Closed ==
  AR_Signal_Solver : nesl_utility/Solver Configuration  PhysicalDomain=network_engine_domain  SubClassName=solver  LeftPortType=input  RightPortType=generic  Tones=[]  Harmonics=[]  SimulateNoise=off  Profile=off  UseLocalSampling=off  EnableSwitchedLinearOptims=on  FrequencyDomain=off  UseCCode=off  RelTol=0.001  AbsTol=0.001  MinStep=1e-09  ToWorkspace=off  RevertToSquareIcSolve=off  NumHomotopyIterations=100  PhasorMode=off  PhasorModeNumHarmonics=1  ConsistencySolver=NEWTON_XTOL_AFTER_FTOL  IndexReductionMethod=DerivativeReplacement  DoDC=off  ResidualTolerance=1e-09  ConsistencyTolSource=GLOBAL  ConsistencyAbsTol=0.001  ConsistencyRelTol=0.001  ConsistencyTolFactor=0.001  UseLocalSolver=off  LocalSolverChoice=NE_BACKWARD_EULER_ADVANCER  ResolveIndetEquations=on  FunctionEvalNumThread=1  LocalSolverSampleTime=0.001  DoFixedCost=off  MaxNonlinIter=3  MaxModeIter=2  ComputeImpulses=off  ImpulseIterations=2  LinearAlgebra=auto  LinearAlgebraNumThread=0  EquationFormulation=NE_TIME_EF  DelaysMemoryBudget=1024  AutomaticFiltering=on  FilteringTimeConstant=0.001  PartitionStorageMethod=AS_NEEDED  PartitionMemoryBudget=1024  PartitionMethod=ROBUST  MultibodyUseLocalSolver=off  MultibodyLocalSolverChoice=ODE1  MultibodyLocalSolverSampleTime=0.001
  AR_Terminator : fl_lib/Physical Signals/Sinks/PS Terminator
  InfiniteFlowResistance : FuelCell_lib/elements/Infinite Flow Resistance (FC)  p_specify=off  p_priority=None  p=0 MPa  p_nominal_specify=off  p_nominal_value=1  p_nominal_unit=MPa  T_specify=off  T_priority=None  T=0 K  T_nominal_specify=off  T_nominal_value=1  T_nominal_unit=K  x_i_specify=off  x_i_priority=None  x_i=[0; 0; 0; 0]  x_i_nominal_specify=off  x_i_nominal_value=1  x_i_nominal_unit=1
      settings: InternalSimscapePortConfiguration="{\"Bottom\":[],\"Left\":[{\"id\":\"A\",\"label\":\"A\",\"type\":\"FuelCell.FuelCell\"}],\"Right\":[{\"id\":\"B\",\"label\":\"B\",\"type\":\"FuelCell.FuelCell\"}],\"Top\":[]}"
  B : PMIOPort  Side=Right
  AR : PMIOPort  Port=2  Side=Left
  A : PMIOPort  Port=3  Side=Left
  connections:
  AR/RConn1 -- AR_Signal_Solver/RConn1 -- AR_Terminator/LConn1
  InfiniteFlowResistance/RConn1 -- B/RConn1
  A/RConn1 -- InfiniteFlowResistance/LConn1

== system PEMFuelCellSystem_Cathode_cEGR_Focused_v01/Cathode_Air_cEGR_BOP/EGRValveRestriction/Open ==
  LocalRestriction : FuelCell_lib/elements/Local Restriction (FC)  const_area=false  restriction_area=cegr_valve_area_low m^2  min_area=cegr_valve_open_min_area m^2  max_area=cegr_valve_max_area m^2  area=cegr_pipe_area m^2  Cd=0.64  B_lam=0.999
      settings: InternalSimscapePortConfiguration="{\"Bottom\":[],\"Left\":[{\"id\":\"AR\",\"label\":\"AR\",\"type\":\"input\"},{\"id\":\"A\",\"label\":\"A\",\"type\":\"FuelCell.FuelCell\"}],\"Right\":[{\"id\":\"B\",\"label\":\"B\",\"type\":\"FuelCell.FuelCell\"}],\"Top\":[]}"
  B : PMIOPort  Side=Right
  AR : PMIOPort  Port=2  Side=Left
  A : PMIOPort  Port=3  Side=Left
  connections:
  AR/RConn1 -- LocalRestriction/LConn1
  LocalRestriction/RConn1 -- B/RConn1
  A/RConn1 -- LocalRestriction/LConn2

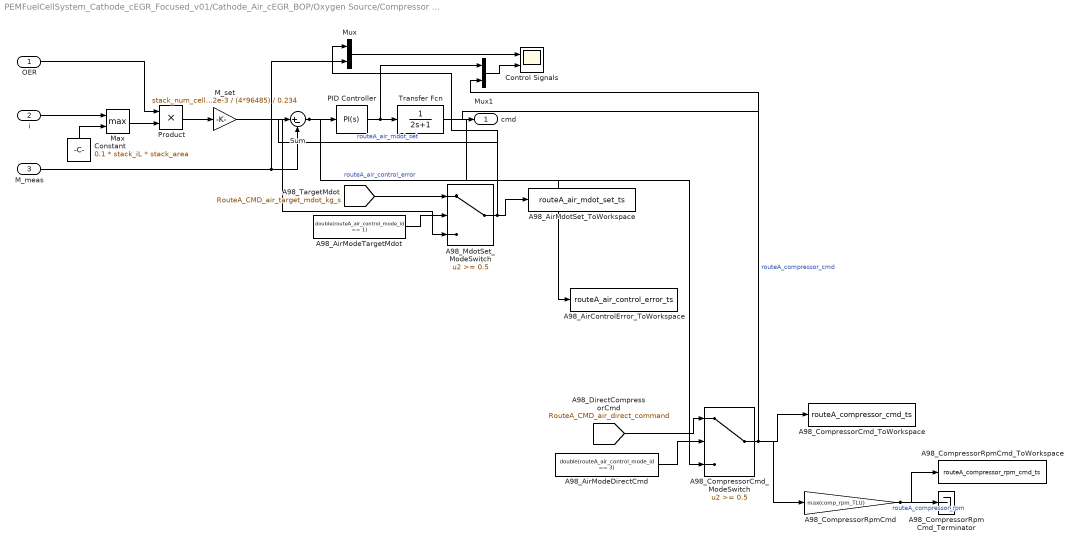
== system PEMFuelCellSystem_Cathode_cEGR_Focused_v01/Cathode_Air_cEGR_BOP/Oxygen Source/Compressor Control ==
  OER : Inport
  i : Inport  Port=2
  M_meas : Inport  Port=3
  A98_AirControlError_ToWorkspace : ToWorkspace  VariableName=routeA_air_control_error_ts  SaveFormat=Timeseries  SampleTime=-1
  A98_AirMdotSet_ToWorkspace : ToWorkspace  VariableName=routeA_air_mdot_set_ts  SaveFormat=Timeseries  SampleTime=-1
  A98_AirModeDirectCmd : Constant  Value=double(routeA_air_control_mode_id == 3)
  A98_AirModeTargetMdot : Constant  Value=double(routeA_air_control_mode_id == 1)
  A98_CompressorCmd_ModeSwitch : Switch  Threshold=0.5  SaturateOnIntegerOverflow=off  InputSameDT=off
  A98_CompressorCmd_ToWorkspace : ToWorkspace  VariableName=routeA_compressor_cmd_ts  SaveFormat=Timeseries  SampleTime=-1
  A98_CompressorRpmCmd : Gain  Gain=max(comp_rpm_TLU)
  A98_CompressorRpmCmd_Terminator : Terminator
  A98_CompressorRpmCmd_ToWorkspace : ToWorkspace  VariableName=routeA_compressor_rpm_cmd_ts  SaveFormat=Timeseries  SampleTime=-1
  A98_MdotSet_ModeSwitch : Switch  Threshold=0.5  SaturateOnIntegerOverflow=off  InputSameDT=off
  Constant : Constant  Value=0.1 * stack_iL * stack_area
  Control Signals : Scope  NumInputPorts=2
      settings: Title=Mass Flow Rate (kg/s)  ActiveDisplayYMinimum=-0.01736  ActiveDisplayYMaximum=0.15625  DataLoggingVariableName=ScopeData2
  M_set : Gain  Gain=stack_num_cells * 32e-3 / (4*96485) / 0.234
  Max : MinMax  Function=max  Inputs=2  ZeroCross=off
  Mux : Mux  Inputs=2
  Mux1 : Mux  Inputs=2
  PID Controller : slpidlib/PID Controller  Controller=PI  Form=Ideal  TimeDomain=Continuous-time  UseExternalTs=off  SampleTime=-1  IntegratorMethod=Forward Euler  FilterMethod=Forward Euler  ControllerParametersSource=internal  P=routeA_air_pid_Kp  I=routeA_air_pid_Ki  UseKiTs=off  D=0  UseExternalDerivativeSource=off  N=100  UseFilter=on  TunerSelectOption=Transfer Function Based (PID Tuner App)  InitialConditionSource=internal  InitialConditionForIntegrator=0  InitialConditionForFilter=0  DifferentiatorICPrevScaledInput=0  ExternalReset=none  TrackingMode=off  Kt=1  LimitOutput=on  SatLimitsSource=internal  UpperSaturationLimit=1  LowerSaturationLimit=0  LinearizeAsGain=on  AntiWindupMode=back-calculation  Kb=1  LimitIntegrator=off  UpperIntegratorSaturationLimit=inf  LowerIntegratorSaturationLimit=-inf  POutMin=[]  POutMax=[]  IOutMin=[]  IOutMax=[]  DOutMin=[]  DOutMax=[]  NOutMin=[]  NOutMax=[]  SumOutMin=[]  SumOutMax=[]  SaturationOutMin=[]  SaturationOutMax=[]  PParamMin=[]  PParamMax=[]  IParamMin=[]  IParamMax=[]  DParamMin=[]  DParamMax=[]  NParamMin=[]  NParamMax=[]  KbParamMin=[]  KbParamMax=[]  KtParamMin=[]  KtParamMax=[]  KbOutMin=[]  KbOutMax=[]  KtOutMin=[]  KtOutMax=[]  IntegratorOutMin=[]  IntegratorOutMax=[]  FilterOutMin=[]  FilterOutMax=[]  SumI1OutMin=[]  SumI1OutMax=[]  SumI2OutMin=[]  SumI2OutMax=[]  SumI3OutMin=[]  SumI3OutMax=[]  SumI4OutMin=[]  SumI4OutMax=[]  SumDOutMin=[]  SumDOutMax=[]  DifferentiatorOutMin=[]  DifferentiatorOutMax=[]  FilterDiffOutCoefMin=[]  FilterDiffOutCoefMax=[]  ReciprocalOutMin=[]  ReciprocalOutMax=[]  SumDenOutMin=[]  SumDenOutMax=[]  SumNumOutMin=[]  SumNumOutMax=[]  DivideOutMin=[]  DivideOutMax=[]  UdiffTsProdOutMin=[]  UdiffTsProdOutMax=[]  NTsProdOutMin=[]  NTsProdOutMax=[]  UintegralTsProdOutMin=[]  UintegralTsProdOutMax=[]  UngainTsProdOutMin=[]  UngainTsProdOutMax=[]  ClampingZeroOutDataTypeStr=Inherit: Inherit via back propagation  ClampingZeroOutMin=[]  ClampingZeroOutMax=[]  FilterDenConstantOutDataTypeStr=Inherit: Inherit via back propagation  FilterDenConstantOutMin=[]  FilterDenConstantOutMax=[]  PCopyOutDataTypeStr=Inherit: Inherit via back propagation  PCopyOutMin=[]  PCopyOutMax=[]  NCopyOutDataTypeStr=Inherit: Inherit via back propagation  NCopyOutMin=[]  NCopyOutMax=[]  IntegratorContinuousStateAttributes=''  IntegratorStateMustResolveToSignalObject=off  IntegratorRTWStateStorageClass=Auto  FilterContinuousStateAttributes=''  FilterStateMustResolveToSignalObject=off  FilterRTWStateStorageClass=Auto  ParallelPVariant=Passthrough  IdealPVariant=InternalParameters  IVariant=InternalParameters  DVariant=Disabled  IntegratorVariant=Continuous  SatVariant=Enabled  AWVariant=BackCalculation  PCopyVariant=Disabled  TRVariant=Disabled  FdbkBlocksVariant=Forward  IdealPFdbkVariant=Disabled  SatFdbkVariant=Disabled  DerivativeFilterVariant=Disabled  NVariant=Disabled  NCopyVariant=Disabled_SignalSpec  FilterICVariant=Disabled  IntegratorICVariant=InternalICs  ExternalResetVariant=Disabled  TRSumVariant=Passthrough  SumFdbkVariant=Disabled  SumVariant=Sum_PI  TsampFilterVariant=InternalTs  TsampNgainVariant=Passthrough  TsampIntegralVariant=Disabled_SignalSpec  ExternalSaturationOutDataTypeStr=Inherit: Same as second input  DerivativeSourceVariant=Disabled  PreIntVariant=InternalPreInt
  Product : Product
  Sum : Sum  Inputs=|+-
  Transfer Fcn : TransferFcn  Denominator=[2 1]
  cmd : Outport
  wires:
  OER/1 -> Product/1
  Constant/1 -> Max/2
  i/1 -> Max/1
  Max/1 -> Product/2
  PID Controller/1 -> Mux1/1, Transfer Fcn/1
  Sum/1 -> PID Controller/1, A98_AirControlError_ToWorkspace/1  "routeA_air_control_error"
  Product/1 -> M_set/1
  M_meas/1 -> Mux/2, Sum/2
  Mux/1 -> Control Signals/1
  Mux1/1 -> Control Signals/2
  A98_AirModeTargetMdot/1 -> A98_MdotSet_ModeSwitch/2
  M_set/1 -> A98_MdotSet_ModeSwitch/3
  A98_MdotSet_ModeSwitch/1 -> Sum/1, Mux/1, A98_AirMdotSet_ToWorkspace/1  "routeA_air_mdot_set"
  A98_AirModeDirectCmd/1 -> A98_CompressorCmd_ModeSwitch/2
  Transfer Fcn/1 -> A98_CompressorCmd_ModeSwitch/3
  A98_CompressorCmd_ModeSwitch/1 -> cmd/1, Mux1/2, A98_CompressorRpmCmd/1, A98_CompressorCmd_ToWorkspace/1  "routeA_compressor_cmd"
  A98_CompressorRpmCmd/1 -> A98_CompressorRpmCmd_Terminator/1, A98_CompressorRpmCmd_ToWorkspace/1  "routeA_compressor_rpm"
  [RouteA_CMD_air_target_mdot_kg_s] -> A98_MdotSet_ModeSwitch/1
  [RouteA_CMD_air_direct_command] -> A98_CompressorCmd_ModeSwitch/1

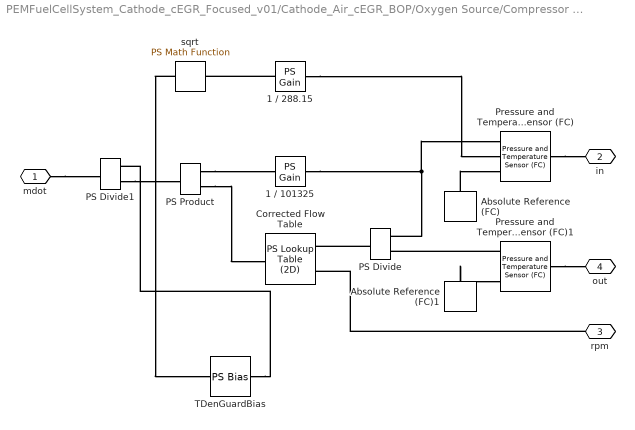
== system PEMFuelCellSystem_Cathode_cEGR_Focused_v01/Cathode_Air_cEGR_BOP/Oxygen Source/Compressor Map ==
  1 / 101325 : fl_lib/Physical Signals/Functions/PS Gain  gain=1 / 101325 1/Pa
  1 / 288.15 : fl_lib/Physical Signals/Functions/PS Gain  gain=1 / 288.15 1/K
  Absolute Reference (FC) : FuelCell_lib/elements/Absolute Reference (FC)
      settings: InternalSimscapePortConfiguration="{\"Bottom\":[],\"Left\":[{\"id\":\"A\",\"label\":\"\",\"type\":\"FuelCell.FuelCell\"}],\"Right\":[],\"Top\":[]}"
  Absolute Reference (FC)1 : FuelCell_lib/elements/Absolute Reference (FC)
      settings: InternalSimscapePortConfiguration="{\"Bottom\":[],\"Left\":[{\"id\":\"A\",\"label\":\"\",\"type\":\"FuelCell.FuelCell\"}],\"Right\":[],\"Top\":[]}"
  Corrected Flow Table : fl_lib/Physical Signals/Lookup Tables/PS Lookup Table (2D)  x1=comp_p_ratio_TLU Pa/Pa  x2=comp_rpm_TLU rpm  f=comp_mdot_corr_TLU kg/s  interp_method=simscape.enum.interpolation.linear  extrap_method=simscape.enum.extrapolation.nearest
  PS Divide : fl_lib/Physical Signals/Functions/PS Divide
  PS Divide1 : fl_lib/Physical Signals/Functions/PS Divide
  PS Product : fl_lib/Physical Signals/Functions/PS Product
  Pressure and Temperature Sensor (FC) : FuelCell_lib/sensors/Pressure and Temperature Sensor (FC)
      settings: InternalSimscapePortConfiguration="{\"Bottom\":[],\"Left\":[{\"id\":\"A\",\"label\":\"A\",\"type\":\"FuelCell.FuelCell\"}],\"Right\":[{\"id\":\"P\",\"label\":\"P\",\"type\":\"output\"},{\"id\":\"T\",\"label\":\"T\",\"type\":\"output\"},{\"id\":\"B\",\"label\":\"B\",\"type\":\"FuelCell.FuelCell\"}],\"Top\":[]}"
  Pressure and Temperature Sensor (FC)1 : FuelCell_lib/sensors/Pressure and Temperature Sensor (FC)
      settings: InternalSimscapePortConfiguration="{\"Bottom\":[],\"Left\":[{\"id\":\"A\",\"label\":\"A\",\"type\":\"FuelCell.FuelCell\"}],\"Right\":[{\"id\":\"P\",\"label\":\"P\",\"type\":\"output\"},{\"id\":\"T\",\"label\":\"T\",\"type\":\"output\"},{\"id\":\"B\",\"label\":\"B\",\"type\":\"FuelCell.FuelCell\"}],\"Top\":[]}"
  TDenGuardBias : fl_lib/Physical Signals/Functions/PS Bias  bias=cegr_comp_map_t_denom_epsilon
      settings: InternalSimscapePortConfiguration="{\"Bottom\":[],\"Left\":[{\"id\":\"I\",\"label\":\"\",\"type\":\"input\"}],\"Right\":[{\"id\":\"O\",\"label\":\"\",\"type\":\"output\"}],\"Top\":[]}"
  sqrt : fl_lib/Physical Signals/Functions/PS Math Function  fcn_choice=foundation.enum.math_function.sqrt  v=1
  mdot : PMIOPort  Side=Left
  in : PMIOPort  Port=2  Side=Right
  rpm : PMIOPort  Port=3  Side=Right
  out : PMIOPort  Port=4  Side=Right
  connections:
  1 / 101325/LConn1 -- Pressure and Temperature Sensor (FC)/RConn1 -- PS Divide/LConn2
  rpm/RConn1 -- Corrected Flow Table/LConn2
  PS Divide/RConn1 -- Corrected Flow Table/LConn1
  1 / 288.15/LConn1 -- Pressure and Temperature Sensor (FC)/RConn2
  PS Product/LConn1 -- 1 / 101325/RConn1
  PS Product/LConn2 -- Corrected Flow Table/RConn1
  PS Divide1/LConn1 -- PS Product/RConn1
  1 / 288.15/RConn1 -- sqrt/LConn1
  mdot/RConn1 -- PS Divide1/RConn1
  Pressure and Temperature Sensor (FC)1/RConn1 -- PS Divide/LConn1
  Absolute Reference (FC)/LConn1 -- Pressure and Temperature Sensor (FC)/RConn3
  Pressure and Temperature Sensor (FC)/LConn1 -- in/RConn1
  Absolute Reference (FC)1/LConn1 -- Pressure and Temperature Sensor (FC)1/RConn3
  Pressure and Temperature Sensor (FC)1/LConn1 -- out/RConn1
  sqrt/RConn1 -- TDenGuardBias/LConn1
  TDenGuardBias/RConn1 -- PS Divide1/LConn2
